simulink model "doubleMassSpringDamper_AdaptiveControl"  (R2021b)
settings: Solver=FixedStepAuto  StartTime=0.0  StopTime=30  FixedStep=0.001  RelTol=1e-3
undefined symbols (not defined in the file): X, Y, Z
libraries: sm_lib x11, nesl_utility x8
settings Model: Creator=Chris  LastModifiedBy=morle
settings SolverCC: AlgebraicLoopSolver=TrustRegion
settings DebuggingCC: SFMachineParentedDataDiag=warning

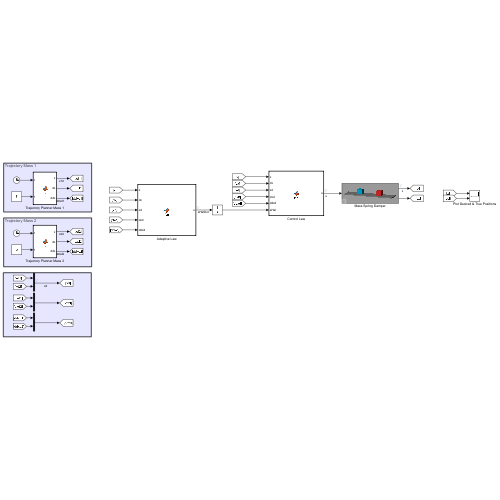
[thumbnail: Simulink's stored preview of the top-level diagram]
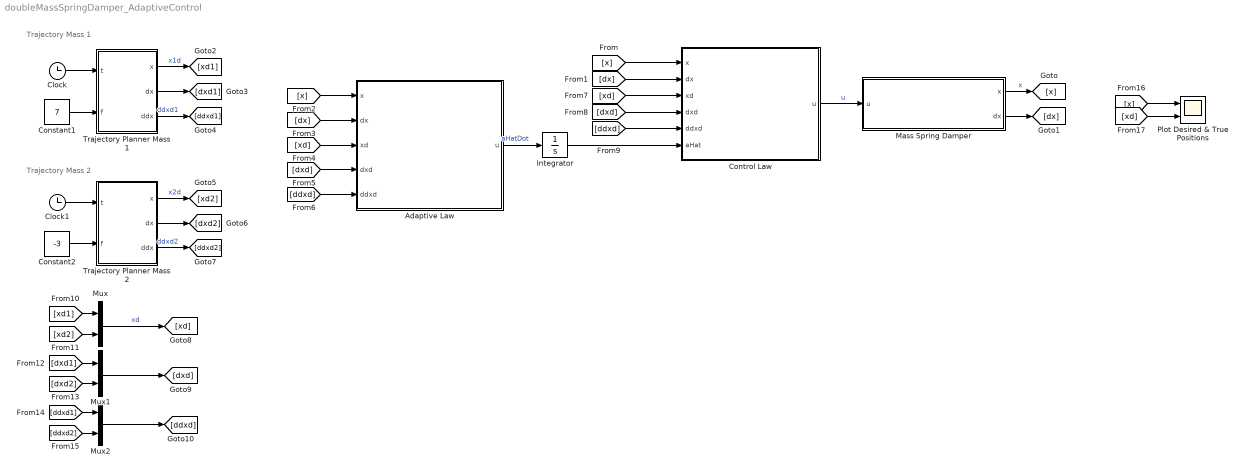
== system doubleMassSpringDamper_AdaptiveControl ==
  note: Trajectory Mass 1
  note: Trajectory Mass 2
  Adaptive Law : MATLAB Function  TreatAsAtomicUnit=on
  Clock : Clock
  Clock1 : Clock
  Constant1 : Constant  Value=7
  Constant2 : Constant  Value=-3
  Control Law : MATLAB Function  TreatAsAtomicUnit=on
  Integrator : Integrator
  Mass Spring Damper : Subsystem  mask{m1=5, m2=60}
      mask prompts: m1 "Mass 1"; m2 "Mass 2"
      mask Display: image('$imagefile'); % Use "Edit Image" on toolstrip to change.
  Mux : Mux  Inputs=2
  Mux1 : Mux  Inputs=2
  Mux2 : Mux  Inputs=2
  Plot Desired & True Positions : Scope  NumInputPorts=2
  Trajectory Planner Mass 1 : MATLAB Function  TreatAsAtomicUnit=on
  Trajectory Planner Mass 2 : MATLAB Function  TreatAsAtomicUnit=on
  wires:
  [x] -> Control Law/1(x)
  [dx] -> Control Law/2(dx)
  Control Law/1(u) -> Mass Spring Damper/1(u)  "u"
  Mass Spring Damper/1(x) -> [x]  "x"
  Mass Spring Damper/2(dx) -> [dx]
  [x] -> Adaptive Law/1(x)
  [dx] -> Adaptive Law/2(dx)
  Trajectory Planner Mass 1/3(ddx) -> [ddxd1]  "ddxd1"
  [xd] -> Adaptive Law/3(xd)
  [dxd] -> Adaptive Law/4(dxd)
  [ddxd] -> Adaptive Law/5(ddxd)
  Adaptive Law/1(u) -> Integrator/1  "aHatDot"
  Integrator/1 -> Control Law/6(aHat)
  [xd] -> Control Law/3(xd)
  [dxd] -> Control Law/4(dxd)
  [ddxd] -> Control Law/5(ddxd)
  Clock1/1 -> Trajectory Planner Mass 2/1(t)
  Trajectory Planner Mass 2/3(ddx) -> [ddxd2]  "ddxd2"
  [xd1] -> Mux/1
  [xd2] -> Mux/2
  Mux/1 -> [xd]  "xd"
  Mux1/1 -> [dxd]
  [dxd2] -> Mux1/2
  [dxd1] -> Mux1/1
  [ddxd1] -> Mux2/1
  [ddxd2] -> Mux2/2
  Mux2/1 -> [ddxd]
  Trajectory Planner Mass 1/1(x) -> [xd1]  "x1d"
  Trajectory Planner Mass 1/2(dx) -> [dxd1]
  Clock/1 -> Trajectory Planner Mass 1/1(t)
  Trajectory Planner Mass 2/2(dx) -> [dxd2]
  Trajectory Planner Mass 2/1(x) -> [xd2]  "x2d"
  Constant1/1 -> Trajectory Planner Mass 1/2(f)
  Constant2/1 -> Trajectory Planner Mass 2/2(f)
  [x] -> Plot Desired & True Positions/1
  [xd] -> Plot Desired & True Positions/2

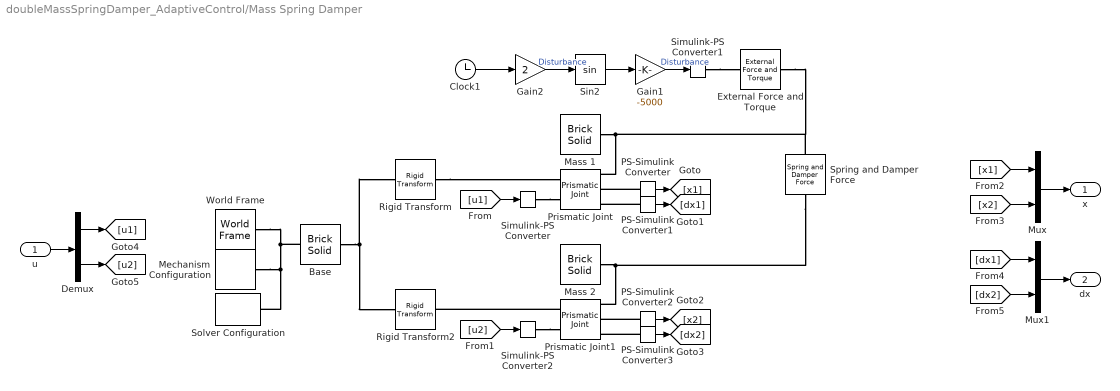
== system doubleMassSpringDamper_AdaptiveControl/Mass Spring Damper ==
  u : Inport
  Base : sm_lib/Body Elements/Brick Solid  GraphicAmbientColor=[0.15 0.15 0.15 1.0]  BasedOnType=Density  BrickDimensions=[10 2 .2]  BrickDimensionUnits=m  CenterOfMass=[0 0 0]  CenterOfMassUnits=m  GraphicDiffuseColor=[0.6 0.6 0.6]  Density=1000  DensityUnits=kg/m^3  DoExposeReferenceFrame=on  GraphicEmissiveColor=[0.0 0.0 0.0 1.0]  ExportEntireGeometry=off  SerializedFrames=<Frames><Frame><Id>Frame1</Id><Value><Name>F1</Name><Origin><Source>ReferenceFrame</Source><FeatureName></FeatureName></Origin><PrimaryAxis><DefinedDirection>+Z</DefinedDirection><Source>ReferenceFrame</Source><SourceDirection>+Z</SourceDirection><FeatureName></FeatureName></PrimaryAxis><SecondaryAxis><DefinedDirection>+X</DefinedDirection><Source>ReferenceFrame</Source><SourceDirection>+X</SourceDirection><FeatureName></FeatureName></SecondaryAxis></Value></Frame></Frames>  MarkerShape=Sphere  MarkerSize=10  GraphicType=FromGeometry  InertiaType=PointMass  Mass=1  MassUnits=kg  MomentsOfInertia=[1 1 1]  MomentsOfInertiaUnits=kg*m^2  GraphicOpacity=1.0  ProductsOfInertia=[0 0 0]  ProductsOfInertiaUnits=kg*m^2  GraphicShininess=75  GraphicSpecularColor=[0.5 0.5 0.5 1.0]  GraphicVisPropType=SimpleVisualProperties
  Clock1 : Clock
  Demux : Demux  Outputs=2
  External Force and Torque : sm_lib/Forces and Torques/External Force and Torque  ForceResolutionFrame=World  EnableForceX=on  EnableForceY=off  EnableForceZ=off  EnableForce=off  TorqueResolutionFrame=AttachedFrame  EnableTorqueX=off  EnableTorqueY=off  EnableTorqueZ=off  EnableTorque=off
  Gain1 : Gain  Gain=-5000
  Gain2 : Gain  Gain=2
  Mass 1 : sm_lib/Body Elements/Brick Solid  GraphicAmbientColor=[0.15 0.15 0.15 1.0]  BasedOnType=Density  BrickDimensions=[1 1 1]  BrickDimensionUnits=m  CenterOfMass=[0 0 0]  CenterOfMassUnits=m  GraphicDiffuseColor=[0.0 0.8 1.0]  Density=1000  DensityUnits=kg/m^3  DoExposeReferenceFrame=on  GraphicEmissiveColor=[0.0 0.0 0.0 1.0]  ExportEntireGeometry=off  SerializedFrames=<Frames/>  MarkerShape=Sphere  MarkerSize=10  GraphicType=FromGeometry  InertiaType=PointMass  Mass=m1  MassUnits=kg  MomentsOfInertia=[1 1 1]  MomentsOfInertiaUnits=kg*m^2  GraphicOpacity=1.0  ProductsOfInertia=[0 0 0]  ProductsOfInertiaUnits=kg*m^2  GraphicShininess=75  GraphicSpecularColor=[0.5 0.5 0.5 1.0]  GraphicVisPropType=SimpleVisualProperties
  Mass 2 : sm_lib/Body Elements/Brick Solid  GraphicAmbientColor=[0.15 0.15 0.15 1.0]  BasedOnType=Density  BrickDimensions=[1 1 1]  BrickDimensionUnits=m  CenterOfMass=[0 0 0]  CenterOfMassUnits=m  GraphicDiffuseColor=[1.0 0.2 0.2]  Density=1000  DensityUnits=kg/m^3  DoExposeReferenceFrame=on  GraphicEmissiveColor=[0.0 0.0 0.0 1.0]  ExportEntireGeometry=off  SerializedFrames=<Frames/>  MarkerShape=Sphere  MarkerSize=10  GraphicType=FromGeometry  InertiaType=PointMass  Mass=m2  MassUnits=kg  MomentsOfInertia=[1 1 1]  MomentsOfInertiaUnits=kg*m^2  GraphicOpacity=1.0  ProductsOfInertia=[0 0 0]  ProductsOfInertiaUnits=kg*m^2  GraphicShininess=75  GraphicSpecularColor=[0.5 0.5 0.5 1.0]  GraphicVisPropType=SimpleVisualProperties
  Mechanism Configuration : sm_lib/Utilities/Mechanism Configuration  UniformGravity=Constant  GravityVector=[0 0 -9.80665]  GravityUnits=m/s^2  LinearizationDelta=0.001  JointModeTransitionNonlinearIterations=2
  Mux : Mux  Inputs=2
  Mux1 : Mux  Inputs=2
  PS-Simulink Converter : nesl_utility/PS-Simulink Converter  PhysicalDomain=network_engine_domain  SubClassName=ps_output  LeftPortType=input  RightPortType=output  PseudoPeriodic=off  Frequencies=[]  Unit=m  AffineConversion=off
      settings: SourceProductBaseCode=PW,SS
  PS-Simulink Converter1 : nesl_utility/PS-Simulink Converter  PhysicalDomain=network_engine_domain  SubClassName=ps_output  LeftPortType=input  RightPortType=output  PseudoPeriodic=off  Frequencies=[]  Unit=m/s  AffineConversion=off
      settings: SourceProductBaseCode=PW,SS
  PS-Simulink Converter2 : nesl_utility/PS-Simulink Converter  PhysicalDomain=network_engine_domain  SubClassName=ps_output  LeftPortType=input  RightPortType=output  PseudoPeriodic=off  Frequencies=[]  Unit=m  AffineConversion=off
      settings: SourceProductBaseCode=PW,SS
  PS-Simulink Converter3 : nesl_utility/PS-Simulink Converter  PhysicalDomain=network_engine_domain  SubClassName=ps_output  LeftPortType=input  RightPortType=output  PseudoPeriodic=off  Frequencies=[]  Unit=m/s  AffineConversion=off
      settings: SourceProductBaseCode=PW,SS
  Prismatic Joint : sm_lib/Joints/Prismatic Joint  JointMode=Normal  SenseConstraintForce=off  SenseConstraintForceX=off  SenseConstraintForceY=off  SenseConstraintForceZ=off  SenseConstraintTorque=off  SenseConstraintTorqueX=off  SenseConstraintTorqueY=off  SenseConstraintTorqueZ=off  SenseTotalForce=off  SenseTotalForceX=off  SenseTotalForceY=off  SenseTotalForceZ=off  SenseTotalTorque=off  SenseTotalTorqueX=off  SenseTotalTorqueY=off  SenseTotalTorqueZ=off  CompositeWrenchDir=FollowerOnBase  CompositeWrenchFrame=BaseFrame  EquilibriumPosition=0  EquilibriumPositionUnits=m  SpringStiffness=0  SpringStiffnessUnits=N/m  DampingCoefficient=4  DampingCoefficientUnits=N/(m/s)  TorqueActuationMode=InputTorque  MotionActuationMode=ComputedMotion  SensePosition=on  SenseVelocity=on  SenseAcceleration=off  SenseTorqueForce=off  SenseLowerLimitTorqueForce=off  SenseUpperLimitTorqueForce=off  LowerLimitSpecify=off  LowerLimitBound=-1  LowerLimitBoundUnits=m  LowerLimitStiffness=1e6  LowerLimitStiffnessUnits=N/m  LowerLimitDamping=1e3  LowerLimitDampingUnits=N/(m/s)  LowerLimitTransitionRegionWidth=1e-4  LowerLimitTransitionRegionWidthUnits=m  UpperLimitSpecify=off  UpperLimitBound=1  UpperLimitBoundUnits=m  UpperLimitStiffness=1e6  UpperLimitStiffnessUnits=N/m  UpperLimitDamping=1e3  UpperLimitDampingUnits=N/(m/s)  UpperLimitTransitionRegionWidth=1e-4  UpperLimitTransitionRegionWidthUnits=m  PositionTargetSpecify=off  PositionTargetPriority=High  PositionTargetValue=0  PositionTargetValueUnits=m  VelocityTargetSpecify=off  VelocityTargetPriority=High  VelocityTargetValue=6  VelocityTargetValueUnits=m/s
  Prismatic Joint1 : sm_lib/Joints/Prismatic Joint  JointMode=Normal  SenseConstraintForce=off  SenseConstraintForceX=off  SenseConstraintForceY=off  SenseConstraintForceZ=off  SenseConstraintTorque=off  SenseConstraintTorqueX=off  SenseConstraintTorqueY=off  SenseConstraintTorqueZ=off  SenseTotalForce=off  SenseTotalForceX=off  SenseTotalForceY=off  SenseTotalForceZ=off  SenseTotalTorque=off  SenseTotalTorqueX=off  SenseTotalTorqueY=off  SenseTotalTorqueZ=off  CompositeWrenchDir=FollowerOnBase  CompositeWrenchFrame=BaseFrame  EquilibriumPosition=0  EquilibriumPositionUnits=m  SpringStiffness=0  SpringStiffnessUnits=N/m  DampingCoefficient=4  DampingCoefficientUnits=N/(m/s)  TorqueActuationMode=InputTorque  MotionActuationMode=ComputedMotion  SensePosition=on  SenseVelocity=on  SenseAcceleration=off  SenseTorqueForce=off  SenseLowerLimitTorqueForce=off  SenseUpperLimitTorqueForce=off  LowerLimitSpecify=off  LowerLimitBound=-1  LowerLimitBoundUnits=m  LowerLimitStiffness=1e6  LowerLimitStiffnessUnits=N/m  LowerLimitDamping=1e3  LowerLimitDampingUnits=N/(m/s)  LowerLimitTransitionRegionWidth=1e-4  LowerLimitTransitionRegionWidthUnits=m  UpperLimitSpecify=off  UpperLimitBound=1  UpperLimitBoundUnits=m  UpperLimitStiffness=1e6  UpperLimitStiffnessUnits=N/m  UpperLimitDamping=1e3  UpperLimitDampingUnits=N/(m/s)  UpperLimitTransitionRegionWidth=1e-4  UpperLimitTransitionRegionWidthUnits=m  PositionTargetSpecify=on  PositionTargetPriority=High  PositionTargetValue=0  PositionTargetValueUnits=m  VelocityTargetSpecify=off  VelocityTargetPriority=High  VelocityTargetValue=0  VelocityTargetValueUnits=m/s
  Rigid Transform : sm_lib/Frames and Transforms/Rigid Transform  TranslationMethod=Cartesian  TranslationStandardOffset=0  TranslationLengthUnit=m  TranslationStandardAxis=+Z  TranslationCartesianOffset=[2 0 0.6]  TranslationROffset=0  TranslationROffsetUnits=m  TranslationZOffset=0  TranslationZOffsetUnits=m  TranslationThetaOffset=0  TranslationThetaOffsetUnits=deg  RotationMethod=StandardAxis  RotationAngleUnits=deg  RotationStandardAxis=+Y  RotationAngle=90  RotationArbitraryAxis=[0 0 1]  FollAlignAxisA=+X  BaseAlignAxisA=+Y  FollAlignAxisB=+Y  BaseAlignAxisB=+Z  RotationSequenceAxes=FollowerAxes  RotationSequence=XYX  RotationSequenceAngles=[0 0 0]  RotationSequenceAnglesUnits=deg  RotationMatrix=[1 0 0; 0 1 0; 0 0 1]
  Rigid Transform2 : sm_lib/Frames and Transforms/Rigid Transform  TranslationMethod=Cartesian  TranslationStandardOffset=0  TranslationLengthUnit=m  TranslationStandardAxis=+Z  TranslationCartesianOffset=[-2 0 0.6]  TranslationROffset=0  TranslationROffsetUnits=m  TranslationZOffset=0  TranslationZOffsetUnits=m  TranslationThetaOffset=0  TranslationThetaOffsetUnits=deg  RotationMethod=StandardAxis  RotationAngleUnits=deg  RotationStandardAxis=+Y  RotationAngle=90  RotationArbitraryAxis=[0 0 1]  FollAlignAxisA=+X  BaseAlignAxisA=+Y  FollAlignAxisB=+Y  BaseAlignAxisB=+Z  RotationSequenceAxes=FollowerAxes  RotationSequence=XYX  RotationSequenceAngles=[0 0 0]  RotationSequenceAnglesUnits=deg  RotationMatrix=[1 0 0; 0 1 0; 0 0 1]
  Simulink-PS Converter : nesl_utility/Simulink-PS Converter  PhysicalDomain=network_engine_domain  SubClassName=ps_input  LeftPortType=input  RightPortType=output  PseudoPeriodic=off  Frequencies=[]  NoiseDistribution=none  NoiseParameters=[]  Unit=1  AffineConversion=off  FilteringAndDerivatives=provide  SimscapeFilterOrder=2  InputFilterTimeConstant=0.001  UdotUserProvided=0
      settings: SourceProductBaseCode=PW,SS
  Simulink-PS Converter1 : nesl_utility/Simulink-PS Converter  PhysicalDomain=network_engine_domain  SubClassName=ps_input  LeftPortType=input  RightPortType=output  PseudoPeriodic=off  Frequencies=[]  NoiseDistribution=none  NoiseParameters=[]  Unit=1  AffineConversion=off  FilteringAndDerivatives=provide  SimscapeFilterOrder=1  InputFilterTimeConstant=0.001  UdotUserProvided=0
      settings: SourceProductBaseCode=PW,SS
  Simulink-PS Converter2 : nesl_utility/Simulink-PS Converter  PhysicalDomain=network_engine_domain  SubClassName=ps_input  LeftPortType=input  RightPortType=output  PseudoPeriodic=off  Frequencies=[]  NoiseDistribution=none  NoiseParameters=[]  Unit=1  AffineConversion=off  FilteringAndDerivatives=provide  SimscapeFilterOrder=2  InputFilterTimeConstant=0.001  UdotUserProvided=0
      settings: SourceProductBaseCode=PW,SS
  Sin2 : Trigonometry
  Solver Configuration : nesl_utility/Solver Configuration  PhysicalDomain=network_engine_domain  SubClassName=solver  LeftPortType=input  RightPortType=generic  Tones=[]  Harmonics=[]  SimulateNoise=off  Profile=off  UseLocalSampling=off  EnableSwitchedLinearOptims=on  FrequencyDomain=off  UseCCode=off  RelTol=0.001  AbsTol=1e-06  MinStep=1e-09  ToWorkspace=off  RevertToSquareIcSolve=off  NumHomotopyIterations=100  PhasorMode=off  PhasorModeNumHarmonics=1  DoDC=off  ResidualTolerance=1e-09  UseLocalSolver=off  LocalSolverChoice=NE_BACKWARD_EULER_ADVANCER  LocalSolverSampleTime=0.001  DoFixedCost=off  MaxNonlinIter=3  MaxModeIter=2  ComputeImpulses=off  ImpulseIterations=2  LinearAlgebra=auto  EquationFormulation=NE_TIME_EF  DelaysMemoryBudget=1024  AutomaticFiltering=on  FilteringTimeConstant=0.001  PartitionStorageMethod=AS_NEEDED  PartitionMemoryBudget=1024  PartitionMethod=ROBUST
      settings: SourceProductBaseCode=PW,SS
  Spring and Damper Force : sm_lib/Forces and Torques/Spring and Damper Force  NaturalLength=4  NaturalLengthUnits=m  SpringStiffness=100  SpringStiffnessUnits=N/m  DampingCoefficient=2  DampingCoefficientUnits=N/(m/s)  SenseForce=off
  World Frame : sm_lib/Frames and Transforms/World Frame
  x : Outport
  dx : Outport  Port=2
  wires:
  Sin2/1 -> Gain1/1
  Clock1/1 -> Gain2/1
  Gain1/1 -> Simulink-PS Converter1/1  "Disturbance"
  Gain2/1 -> Sin2/1  "Disturbance"
  Mux/1 -> x/1
  Mux1/1 -> dx/1
  PS-Simulink Converter/1 -> [x1]
  PS-Simulink Converter1/1 -> [dx1]
  PS-Simulink Converter2/1 -> [x2]
  PS-Simulink Converter3/1 -> [dx2]
  [u2] -> Simulink-PS Converter2/1
  u/1 -> Demux/1
  Demux/1 -> [u1]
  Demux/2 -> [u2]
  [x1] -> Mux/1
  [x2] -> Mux/2
  [dx1] -> Mux1/1
  [dx2] -> Mux1/2
  [u1] -> Simulink-PS Converter/1
  connections:
  World Frame/RConn1 -- Solver Configuration/RConn1 -- Mechanism Configuration/RConn1 -- Base/RConn1
  Mass 1/RConn1 -- Prismatic Joint/RConn1 -- Spring and Damper Force/LConn1 -- External Force and Torque/RConn1
  Rigid Transform/RConn1 -- Prismatic Joint/LConn1
  PS-Simulink Converter1/LConn1 -- Prismatic Joint/RConn3
  Simulink-PS Converter/RConn1 -- Prismatic Joint/LConn2
  PS-Simulink Converter/LConn1 -- Prismatic Joint/RConn2
  Base/LConn1 -- Rigid Transform2/LConn1 -- Rigid Transform/LConn1
  Mass 2/RConn1 -- Spring and Damper Force/RConn1 -- Prismatic Joint1/RConn1
  Simulink-PS Converter2/RConn1 -- Prismatic Joint1/LConn2
  PS-Simulink Converter3/LConn1 -- Prismatic Joint1/RConn3
  PS-Simulink Converter2/LConn1 -- Prismatic Joint1/RConn2
  Prismatic Joint1/LConn1 -- Rigid Transform2/RConn1
  Simulink-PS Converter1/RConn1 -- External Force and Torque/LConn1

== matlab function doubleMassSpringDamper_AdaptiveControl/Adaptive Law ==
  data: x input; u output; dx input; xd input; dxd input; ddxd input
function u  = fcn(x,dx,xd,dxd,ddxd)
%Demux the incoming variables
x1=x(1);
x2=x(2);

dx1=dx(1);
dx2=dx(2);

x1d=xd(1);
x2d=xd(2);

dx1d=dxd(1);
dx2d=dxd(2);

ddx1d=ddxd(1);
ddx2d=ddxd(2);

%Define constants that appear in the control law
P=10;
lambda=-20*eye(2);

%Define the error terms
xError=[x1-x1d;x2-x2d];
dxError=[dx1-dx1d;dx2-dx2d];

%Define all the qr terms
dxr=dxd+lambda*xError;
ddxr=ddxd+lambda*dxError;

%Define S
S=dxError-lambda*xError;

%Define Y
Y=[(x1-x2) , dxr(1) , -dxr(2) , ddxr(1) , 0 , 0 ;(-x1+x2) , 0 , -dxr(1) , 0 , dxr(2) , ddxr(2)];

u=-P*transpose(Y)*S;

== matlab function doubleMassSpringDamper_AdaptiveControl/Control Law ==
  data: x input; u output; dx input; xd input; dxd input; ddxd input; aHat input
function u  = fcn(x,dx,xd,dxd,ddxd,aHat)
%Demux the incoming variables
x1=x(1);
x2=x(2);

dx1=dx(1);
dx2=dx(2);

x1d=xd(1);
x2d=xd(2);

dx1d=dxd(1);
dx2d=dxd(2);

ddx1d=ddxd(1);
ddx2d=ddxd(2);

%Define the error terms
xError=(x-xd);
dxError=(dx-dxd);

%Define constants that appear in the control law
lambda=-100*eye(2);
K=[1000 0;0 1000];

%Define all the qr terms
dxr=dxd+lambda*xError;
ddxr=ddxd+lambda*dxError;

%Define Y
Y=[(x1-x2) , dxr(1) , -dxr(2) , ddxr(1) , 0 , 0 ;(-x1+x2) , 0 , -dxr(1) , 0 , dxr(2) , ddxr(2)];

%Define Hyperplane
S=dxError-lambda*xError;


u=Y*aHat-K*S;

== matlab function doubleMassSpringDamper_AdaptiveControl/Trajectory Planner Mass 1 ==
  data: t input; x output; f input; dx output; ddx output
function [x,dx,ddx] = fcn(t,f)

x=sin(f*t);
dx=f*cos(f*t);
ddx=-f^2*sin(f*t);

== matlab function doubleMassSpringDamper_AdaptiveControl/Trajectory Planner Mass 2 ==
  data: t input; x output; f input; dx output; ddx output
function [x,dx,ddx] = fcn(t,f)

x=sin(f*t);
dx=f*cos(f*t);
ddx=-f^2*sin(f*t);
